simulink model "ame532Project1_Gimbal_Tracking_R2022aVersion_JeosUpdates"  (R2022a)
settings: Solver=ode4  StartTime=0.0  StopTime=35  FixedStep=0.1  RelTol=1e-3
model workspace (MAT data in the model file):
  theta : Simulink.Parameter (value not decoded)
values from neighbouring files (symbols this model uses):
  a0_s2 = 0    [AeroData.m]
  a0_s3 = 0    [AeroData.m]
  a0_s4 = 0.05    [AeroData.m]
  a0_s5 = 0.05    [AeroData.m]
  CD0_s2 = 0.01    [AeroData.m]
  CD0_s3 = 0.01    [AeroData.m]
  CD0_s4 = 0.01    [AeroData.m]
  CD0_s5 = 0.01    [AeroData.m]
  CDa_s2 = 1    [AeroData.m]
  CDa_s3 = 1    [AeroData.m]
  CDa_s4 = 1    [AeroData.m]
  CDa_s5 = 1    [AeroData.m]
  CL0_s2 = 0    [AeroData.m]
  CL0_s3 = 0    [AeroData.m]
  CL0_s4 = 0.05    [AeroData.m]
  CL0_s5 = 0.05    [AeroData.m]
  CM0_s2 = 0    [AeroData.m]
  CM0_s3 = 0    [AeroData.m]
  CM0_s4 = -0.05    [AeroData.m]
  CM0_s5 = -0.05    [AeroData.m]
  CMa_s2 = 0    [AeroData.m]
  CMa_s3 = 0    [AeroData.m]
  CMa_s4 = 0    [AeroData.m]
  CMa_s5 = 0    [AeroData.m]
  e_s2 = 0.8    [AeroData.m]
  e_s3 = 0.8    [AeroData.m]
  e_s4 = 0.9    [AeroData.m]
  e_s5 = 0.9    [AeroData.m]
  i_s2 = 0    [AeroData.m]
  i_s3 = 0    [AeroData.m]
  i_s4 = 0.05    [AeroData.m]
  i_s5 = 0.05    [AeroData.m]
  Jxx = 1    [Sim_sixDOFdriverScript.m]
  Jxy = 0.    (= 0)    [Sim_sixDOFdriverScript.m]
  Jxz = 3    [Sim_sixDOFdriverScript.m]
  Jyx = 2    [Sim_sixDOFdriverScript.m]
  Jyy = 2    [Sim_sixDOFdriverScript.m]
  Jyz = 0    [Sim_sixDOFdriverScript.m]
  Jzx = Jxz    (= 3)    [Sim_sixDOFdriverScript.m]
  Jzy = Jyz    (= 0)    [Sim_sixDOFdriverScript.m]
  Jzz = 2    [Sim_sixDOFdriverScript.m]
  LL = 0.8    [Sim_sixDOFdriverScript.m]
  MM = 0.8    [Sim_sixDOFdriverScript.m]
  n_s2 = [0; 0; -1]    [AeroData.m]
  n_s3 = [0; 1; 0]    [AeroData.m]
  n_s4 = [0; 0; -1]    [AeroData.m]
  n_s5 = [0; 0; -1]    [AeroData.m]
  NN = 0.8    [Sim_sixDOFdriverScript.m]
  rEarth = 6378100    [Sim_sixDOFdriverScript.m]
  ro = 1.225    [AeroData.m]
undefined symbols (not defined in the file or in its folder): AR_s2, AR_s3, AR_s4, AR_s5, area_s2, area_s3, area_s4, area_s5, c_s2, c_s3, c_s4, c_s5, earthRadius, x_S2_B_B, x_S3_B_B, x_S4_B_B, x_S5_B_B
libraries: simulink_extras x37, matrix_library x21, aerolibutil x6, aerolibfltsims x4, simulink x3, vrlib x2, aerolibtransform2 x2, sharedutil x2
(part 2 of 5)

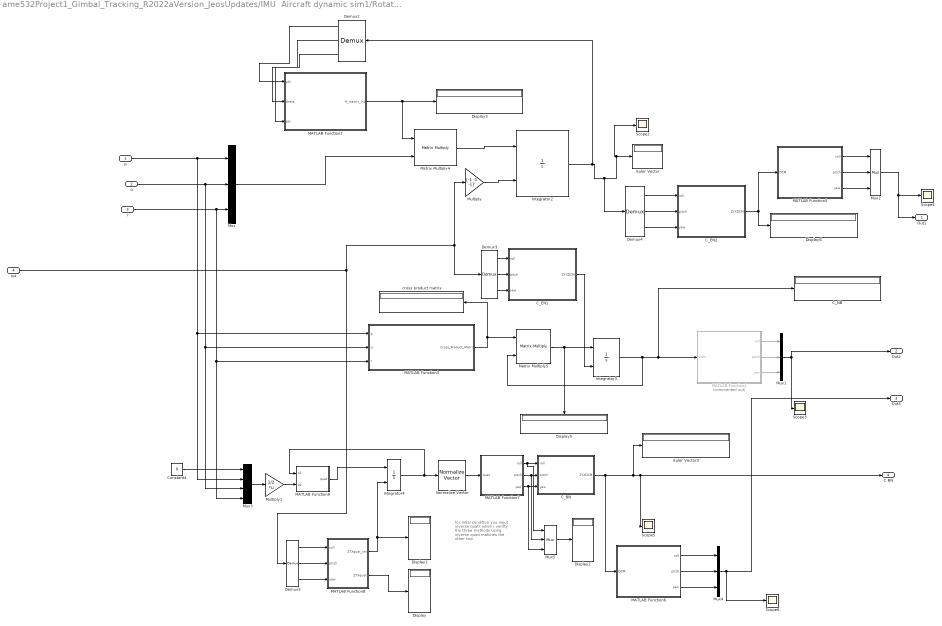
== system ame532Project1_Gimbal_Tracking_R2022aVersion_JeosUpdates/IMU  Aircraft dynamic sim1/Rotational Kinematics ==
  note: for intial condition you input inverse quat?
      | when I verifty the three methods using inverse quad matches the other two
  p : Inport
  q : Inport  Port=2
  r : Inport  Port=3
  In4 : Inport  Port=4
  C_BN : MATLAB Function  TreatAsAtomicUnit=on
  C_EN1 : MATLAB Function  TreatAsAtomicUnit=on
  C_EN2 : MATLAB Function  TreatAsAtomicUnit=on
  C_NB : Display
  Constant4 : Constant  Value=0
  Demux{2..5} (4 alike) : Demux  Outputs=3
  Display{,1..3,5..6} (6 alike) : Display
  Euler Vector : Display
  Euler Vector3 : Display
  Integrator2 : Integrator  InitialConditionSource=external
  Integrator3 : Integrator  InitialConditionSource=external
  Integrator4 : Integrator  InitialConditionSource=external  InitialCondition=[1 0 0 0]'
  MATLAB Function2 : MATLAB Function  TreatAsAtomicUnit=on
  MATLAB Function3 : MATLAB Function  TreatAsAtomicUnit=on
  MATLAB Function4 : MATLAB Function  Commented=on  TreatAsAtomicUnit=on
  MATLAB Function5 : MATLAB Function  TreatAsAtomicUnit=on
  MATLAB Function6 : MATLAB Function  TreatAsAtomicUnit=on
  MATLAB Function7 : MATLAB Function  TreatAsAtomicUnit=on
  MATLAB Function8 : MATLAB Function  TreatAsAtomicUnit=on
  MATLAB Function9 : MATLAB Function  TreatAsAtomicUnit=on
  Matrix Multiply4 : Product  Multiplication=Matrix(*)
  Matrix Multiply5 : Product  Multiplication=Matrix(*)
  Multiply : Gain  Gain=[-1 -1 -1]'
  Multiply1 : Gain  Gain=1/2  Multiplication=Matrix(K*u)
  Mux{,1..2,4..5} (5 alike) : Mux  Inputs=3
  Mux3 : Mux
  Normalize Vector : vrlib/Utilities/Normalize Vector  maxzero=0
  Scope{2..6} (5 alike) : Scope
  cross product matrix : Display
  Out1 : Outport
  Out2 : Outport  Port=2
  Out3 : Outport  Port=3
  C BN : Outport  Port=4
  wires:
  Matrix Multiply4/1 -> Integrator2/1
  In4/1 -> Multiply/1, Demux3/1, Demux5/1
  MATLAB Function4/3(yaw) -> Mux1/3
  Integrator2/1 -> Scope2/1, Euler Vector/1, Demux4/1, Demux2/1
  MATLAB Function2/1(H_matrix_inv) -> Display3/1, Matrix Multiply4/1
  MATLAB Function6/2(pitch) -> Mux4/2
  r/1 -> Mux3/4, MATLAB Function3/3(r), Mux/3
  Matrix Multiply5/1 -> Display5/1, Integrator3/1
  Mux/1 -> Matrix Multiply4/2
  q/1 -> Mux3/3, MATLAB Function3/2(q), Mux/2
  C_BN/1(ZYXDCM) -> MATLAB Function6/1(DCM), C BN/1, Scope5/1, Euler Vector3/1
  C_EN1/1(ZYXDCM) -> Integrator3/2
  MATLAB Function5/2(pitch) -> Mux2/2
  Mux1/1 -> Out2/1, Scope3/1
  MATLAB Function4/1(roll) -> Mux1/1
  Demux2/2 -> MATLAB Function2/2(theta)
  Demux4/3 -> C_EN2/3(yaw)
  MATLAB Function4/2(pitch) -> Mux1/2
  Demux2/3 -> MATLAB Function2/3(psi)
  Demux2/1 -> MATLAB Function2/1(phi)
  Demux5/1 -> MATLAB Function8/1(roll)
  Demux3/1 -> C_EN1/1(roll)
  Demux5/2 -> MATLAB Function8/2(pitch)
  Demux4/1 -> C_EN2/1(roll)
  Demux3/3 -> C_EN1/3(yaw)
  Multiply/1 -> Integrator2/2
  C_EN2/1(ZYXDCM) -> Display6/1, MATLAB Function5/1(DCM)
  Normalize Vector/1 -> MATLAB Function7/1(quat)
  MATLAB Function9/1(quat) -> Integrator4/1
  Integrator3/1 -> Matrix Multiply5/2, MATLAB Function4/1(DCM), C_NB/1
  p/1 -> Mux3/2, MATLAB Function3/1(p), Mux/1
  Integrator4/1 -> Normalize Vector/1, MATLAB Function9/1(q1)
  MATLAB Function7/3(yaw) -> Mux5/3, C_BN/3(yaw)
  Mux2/1 -> Out1/1, Scope4/1
  MATLAB Function5/3(yaw) -> Mux2/3
  Constant4/1 -> Mux3/1
  Mux3/1 -> Multiply1/1
  Mux4/1 -> Out3/1, Scope6/1
  MATLAB Function7/1(roll) -> Mux5/1, C_BN/1(roll)
  MATLAB Function5/1(roll) -> Mux2/1
  Demux5/3 -> MATLAB Function8/3(yaw)
  MATLAB Function6/1(roll) -> Mux4/1
  MATLAB Function6/3(yaw) -> Mux4/3
  Multiply1/1 -> MATLAB Function9/2(q2)
  MATLAB Function3/1(Cross_Product_Matrix) -> Matrix Multiply5/1, cross product matrix/1
  Demux4/2 -> C_EN2/2(pitch)
  Demux3/2 -> C_EN1/2(pitch)
  MATLAB Function7/2(pitch) -> Mux5/2, C_BN/2(pitch)
  MATLAB Function8/1(ZYXquat_inv) -> Integrator4/2, Display1/1
  MATLAB Function8/2(ZYXquat) -> Display/1
  Mux5/1 -> Display2/1

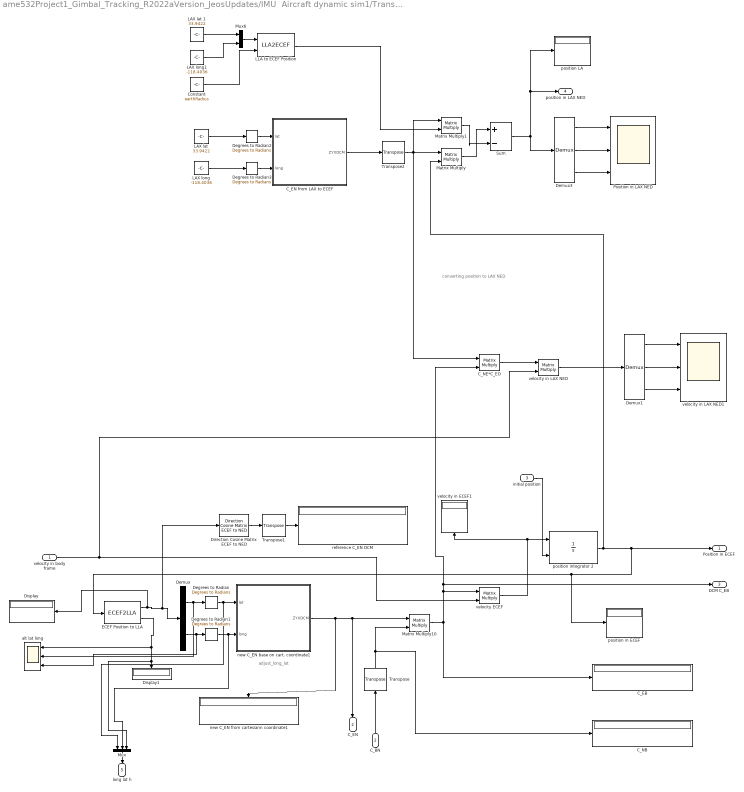
== system ame532Project1_Gimbal_Tracking_R2022aVersion_JeosUpdates/IMU  Aircraft dynamic sim1/Translational Kinematics ==
  note: converting position to LAX NED
  note: adjust_long_lat
  velocity in body frame : Inport
  C_BN : Inport  Port=2
  initial position : Inport  Port=3
  C_EB : Display
  C_EN from LAX to ECEF : MATLAB Function  TreatAsAtomicUnit=on
  C_NB : Display
  C_NE*C_EO : Product  Multiplication=Matrix(*)
  Constant : Constant  Value=earthRadius
  Degrees to Radian{,1..3} (4 alike) : simulink_extras/Transformations/Degrees to Radians
  Demux : Demux  Outputs=2
  Demux1 : Demux  Outputs=3
  Demux3 : Demux  Outputs=3
  Direction Cosine Matrix ECEF to NED : aerolibtransform2/Direction Cosine Matrix ECEF to NED
  Display : Display
  Display1 : Display
  ECEF Position to LLA : ECEF2LLA  ptype=Custom  R=earthRadius
  "LAX lat " : Constant  Value=33.9422
  LAX lat 1 : Constant  Value=33.9422
  LAX long : Constant  Value=-118.4036
  LAX long1 : Constant  Value=-118.4036
  LLA to ECEF Position : LLA2ECEF
  Matrix Multiply : Product  Multiplication=Matrix(*)
  Matrix Multiply1 : Product  Multiplication=Matrix(*)
  Matrix Multiply10 : Product  Multiplication=Matrix(*)
  Mux : Mux  Inputs=3
  Mux6 : Mux  Inputs=2
  Position in LAX NED : Scope  NumInputPorts=3
  Sum : Sum  Inputs=|+-
  Transpose : matrix_library/Transpose
  Transpose1 : matrix_library/Transpose
  Transpose2 : matrix_library/Transpose
  alt lat long : Scope  NumInputPorts=3
  new C_EN base on cart. coordinate1 : MATLAB Function  TreatAsAtomicUnit=on
  new C_EN from cartesiann coordinate1 : Display
  "position LA " : Display
  position in ECEF : Display
  position integrator 2 : Integrator  InitialConditionSource=external  InitialCondition=[6378100,0,0]'
  reference C_EN DCM : Display
  velocity ECEF : Product  Multiplication=Matrix(*)
  velocity in ECEF1 : Display
  velocity in LAX NED : Product  Multiplication=Matrix(*)
  velocity in LAX NED1 : Scope  NumInputPorts=3
  Position in ECEF : Outport
  C_EN : Outport  Port=2
  DCM C_EB : Outport  Port=3
  position in LAX NED : Outport  Port=4
  long lat h : Outport  Port=5
  wires:
  initial position/1 -> position integrator 2/2
  new C_EN base on cart. coordinate1/1(ZYXDCM) -> new C_EN from cartesiann coordinate1/1, C_EN/1, Matrix Multiply10/1
  Matrix Multiply10/1 -> C_EB/1, DCM C_EB/1, C_NE*C_EO/2, velocity ECEF/1
  velocity ECEF/1 -> position integrator 2/1, velocity in ECEF1/1
  velocity in body frame/1 -> velocity in LAX NED/2, velocity ECEF/2
  C_BN/1 -> Transpose/1
  ECEF Position to LLA/1 -> Direction Cosine Matrix ECEF to NED/1, Demux/1, Display/1
  ECEF Position to LLA/2 -> alt lat long/1, Mux/3, Display1/1
  Demux/1 -> Degrees to Radian/1, alt lat long/2
  Demux/2 -> alt lat long/3, Degrees to Radian1/1
  Degrees to Radian/1 -> Mux/1, new C_EN base on cart. coordinate1/1(lat)
  Degrees to Radian1/1 -> Mux/2, new C_EN base on cart. coordinate1/2(long)
  Transpose/1 -> C_NB/1, Matrix Multiply10/2
  Direction Cosine Matrix ECEF to NED/1 -> Transpose1/1
  Transpose1/1 -> reference C_EN DCM/1
  Mux/1 -> long lat h/1
  "LAX lat "/1 -> Degrees to Radian2/1
  LAX long/1 -> Degrees to Radian3/1
  Degrees to Radian2/1 -> C_EN from LAX to ECEF/1(lat)
  Degrees to Radian3/1 -> C_EN from LAX to ECEF/2(long)
  C_EN from LAX to ECEF/1(ZYXDCM) -> Transpose2/1
  Demux3/2 -> Position in LAX NED/2
  Demux3/3 -> Position in LAX NED/3
  Demux3/1 -> Position in LAX NED/1
  Transpose2/1 -> C_NE*C_EO/1, Matrix Multiply1/1, Matrix Multiply/1
  LAX long1/1 -> Mux6/2
  LAX lat 1/1 -> Mux6/1
  Constant/1 -> LLA to ECEF Position/2
  Mux6/1 -> LLA to ECEF Position/1
  LLA to ECEF Position/1 -> Matrix Multiply1/2
  Matrix Multiply/1 -> Sum/1
  Matrix Multiply1/1 -> Sum/2
  Sum/1 -> "position LA "/1, position in LAX NED/1, Demux3/1
  position integrator 2/1 -> Position in ECEF/1, ECEF Position to LLA/1, position in ECEF/1, Matrix Multiply/2
  C_NE*C_EO/1 -> velocity in LAX NED/1
  Demux1/2 -> velocity in LAX NED1/2
  velocity in LAX NED/1 -> Demux1/1
  Demux1/3 -> velocity in LAX NED1/3
  Demux1/1 -> velocity in LAX NED1/1

== system ame532Project1_Gimbal_Tracking_R2022aVersion_JeosUpdates/IMU  Aircraft dynamic sim1/Unused tranlational kinmatics ==
  In1 : Inport
  In2 : Inport  Port=2
  In3 : Inport  Port=3
  C_EN4 : MATLAB Function  TreatAsAtomicUnit=on
  DCM4 : Display
  Matrix Multiply8 : Product  Multiplication=Matrix(*)
  Matrix Multiply9 : Product  Multiplication=Matrix(*)
  Scope7 : Scope
  Transpose : matrix_library/Transpose
  pitch4 : Constant  Value=pi/2
  position integrator 1 : Integrator  InitialConditionSource=external  InitialCondition=[6378100,0,0]'
  position vector2 : Display
  roll4 : Constant  Value=0
  velocity in earth frame : Display
  yaw4 : Constant  Value=0
  wires:
  Matrix Multiply9/1 -> DCM4/1, Matrix Multiply8/1
  position integrator 1/1 -> Scope7/1, position vector2/1
  C_EN4/1(ZYXDCM) -> Matrix Multiply9/1
  Matrix Multiply8/1 -> velocity in earth frame/1, position integrator 1/1
  yaw4/1 -> C_EN4/3(yaw)
  pitch4/1 -> C_EN4/2(pitch)
  Transpose/1 -> Matrix Multiply9/2
  roll4/1 -> C_EN4/1(roll)
  In2/1 -> Matrix Multiply8/2
  In1/1 -> position integrator 1/2
  In3/1 -> Transpose/1

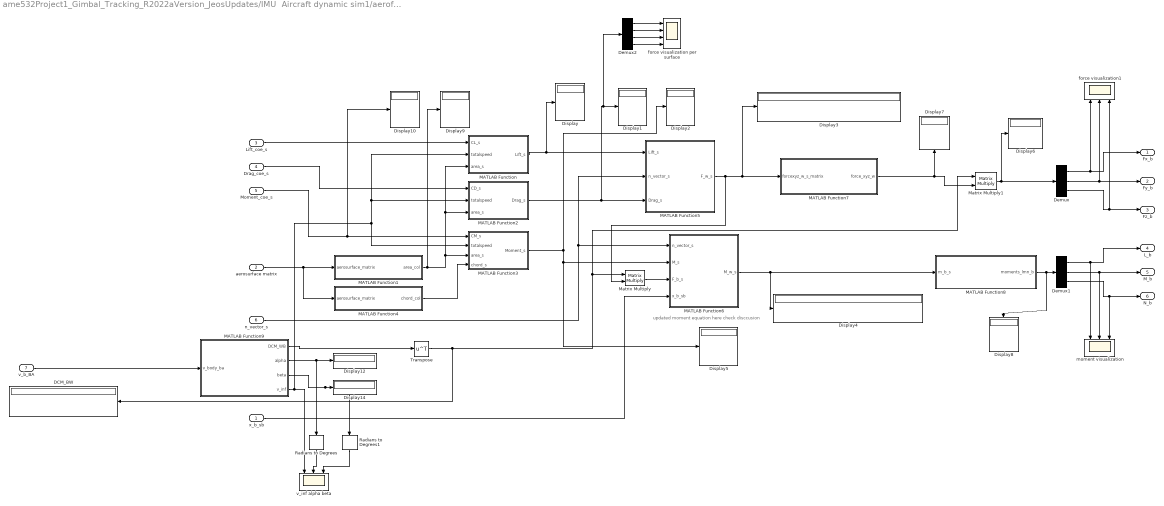
== system ame532Project1_Gimbal_Tracking_R2022aVersion_JeosUpdates/IMU  Aircraft dynamic sim1/aeroforce & moment block ==
  note: updated moment equation here check disccusion
  x_b_sb : Inport
  aerosurface matrix : Inport  Port=2
  Lift_coe_s : Inport  Port=3
  Drag_coe_s : Inport  Port=4
  Moment_coe_s : Inport  Port=5
  n_vector_s : Inport  Port=6
  v_b_BA : Inport  Port=7
  DCM_BW : Display
  Demux : Demux  Outputs=3
  Demux1 : Demux  Outputs=3
  Demux2 : Demux
  Display{,1..10,12,14} (13 alike) : Display
  MATLAB Function : MATLAB Function  TreatAsAtomicUnit=on
  MATLAB Function1 : MATLAB Function  TreatAsAtomicUnit=on
  MATLAB Function2 : MATLAB Function  TreatAsAtomicUnit=on
  MATLAB Function3 : MATLAB Function  TreatAsAtomicUnit=on
  MATLAB Function4 : MATLAB Function  TreatAsAtomicUnit=on
  MATLAB Function5 : MATLAB Function  TreatAsAtomicUnit=on
  MATLAB Function6 : MATLAB Function  TreatAsAtomicUnit=on
  MATLAB Function7 : MATLAB Function  TreatAsAtomicUnit=on
  MATLAB Function8 : MATLAB Function  TreatAsAtomicUnit=on
  MATLAB Function9 : MATLAB Function  TreatAsAtomicUnit=on
  Matrix Multiply : Product  Multiplication=Matrix(*)
  Matrix Multiply1 : Product  Multiplication=Matrix(*)
  Radians to Degrees : simulink_extras/Transformations/Radians to Degrees
  Radians to Degrees1 : simulink_extras/Transformations/Radians to Degrees
  Transpose : Math  Operator=transpose
  force visualization per surface : Scope  NumInputPorts=4
  force visualization1 : Scope  NumInputPorts=3
  moment visualization : Scope  NumInputPorts=3
  v_inf alpha beta : Scope  NumInputPorts=3
  Fx_b : Outport
  Fy_b : Outport  Port=2
  Fz_b : Outport  Port=3
  L_b : Outport  Port=4
  M_b : Outport  Port=5
  N_b : Outport  Port=6
  wires:
  Lift_coe_s/1 -> MATLAB Function/1(CL_s)
  MATLAB Function9/4(v_inf) -> v_inf alpha beta/1, MATLAB Function2/2(totalspeed), MATLAB Function/2(totalspeed), MATLAB Function3/2(totalspeed)
  aerosurface matrix/1 -> MATLAB Function4/1(aerosurface_matrix), MATLAB Function1/1(aerosurface_matrix)
  MATLAB Function1/1(area_col) -> Display9/1, MATLAB Function2/3(area_s), MATLAB Function/3(area_s), MATLAB Function3/3(area_s)
  Drag_coe_s/1 -> MATLAB Function2/1(CD_s)
  Moment_coe_s/1 -> Display10/1, MATLAB Function3/1(CM_s)
  MATLAB Function4/1(chord_col) -> MATLAB Function3/4(chord_s)
  n_vector_s/1 -> MATLAB Function5/2(n_vector_s), MATLAB Function6/1(n_vector_s)
  MATLAB Function/1(Lift_s) -> Display/1, MATLAB Function5/1(Lift_s)
  MATLAB Function2/1(Drag_s) -> MATLAB Function5/3(Drag_s), Demux2/1, Display1/1
  MATLAB Function3/1(Moment_s) -> Display5/1, MATLAB Function6/2(M_s), Display2/1
  MATLAB Function6/1(M_w_s) -> Display4/1, MATLAB Function8/1(m_b_s)
  Matrix Multiply/1 -> MATLAB Function6/3(F_b_s)
  x_b_sb/1 -> MATLAB Function6/4(x_b_sb)
  MATLAB Function5/1(F_w_s) -> Matrix Multiply/2, Display3/1, MATLAB Function7/1(forcexyz_w_s_matrix)
  MATLAB Function7/1(force_xyz_w) -> Matrix Multiply1/2, Display7/1
  MATLAB Function8/1(moments_lmn_b) -> Demux1/1, Display8/1
  Matrix Multiply1/1 -> Demux/1, Display6/1
  MATLAB Function9/1(DCM_WB) -> Transpose/1
  v_b_BA/1 -> MATLAB Function9/1(v_body_ba)
  MATLAB Function9/2(alpha) -> Radians to Degrees/1, Display12/1
  MATLAB Function9/3(beta) -> Display14/1, Radians to Degrees1/1
  Demux1/1 -> L_b/1, moment visualization/1
  Demux1/2 -> M_b/1, moment visualization/2
  Demux1/3 -> moment visualization/3, N_b/1
  Demux/1 -> Fx_b/1, force visualization1/1
  Demux/2 -> Fy_b/1, force visualization1/2
  Demux/3 -> Fz_b/1, force visualization1/3
  Transpose/1 -> Matrix Multiply1/1, Matrix Multiply/1, DCM_BW/1
  Radians to Degrees/1 -> v_inf alpha beta/2
  Radians to Degrees1/1 -> v_inf alpha beta/3
  Demux2/4 -> force visualization per surface/4
  Demux2/3 -> force visualization per surface/3
  Demux2/2 -> force visualization per surface/2
  Demux2/1 -> force visualization per surface/1

== system ame532Project1_Gimbal_Tracking_R2022aVersion_JeosUpdates/IMU  Aircraft dynamic sim1/aeroforce coefficient block ==
  note: next step is to create lift force, CD, CM
  aero surface property matrix : Inport
  real wind in N axes : Inport  Port=2
  velocity in bodyframe : Inport  Port=3
  C_BN : Inport  Port=4
  CD0 : Constant  Value=[0.01 0.01 0.01 0.01]'
  CD1 : Constant  Value=[0.9 0.9 0.8 0.8]'
  CD_a : Constant  Value=[1 1 1 1]'
  CL over time : Scope  NumInputPorts=4
  CL0 : Constant  Value=[0.05 0.05 0 0]'
  CM_0 : Constant  Value=[-0.05 -0.05 0 0]'
  CM_a : Constant  Value=[0 0 0 0]'
  Demux1 : Demux
  Demux5 : Demux
  Demux6 : Demux  Outputs=3
  Display{,1..3,5..7} (7 alike) : Display
  MATLAB Function : MATLAB Function  TreatAsAtomicUnit=on
  MATLAB Function1 : MATLAB Function  TreatAsAtomicUnit=on
  MATLAB Function2 : MATLAB Function  TreatAsAtomicUnit=on
  MATLAB Function3 : MATLAB Function  TreatAsAtomicUnit=on
  alpha : Scope  NumInputPorts=4
  alpha_0 : Constant  Value=[0.05 0.05 0 0]'
  calculatie alpha : MATLAB Function  TreatAsAtomicUnit=on
  extract matrix function : MATLAB Function  TreatAsAtomicUnit=on
  extract matrix function1 : MATLAB Function  TreatAsAtomicUnit=on
  i0 : Constant  Value=[0.05 0.05 0 0]'
  n vector(4 5 2 3 from left to right) : Constant  Value=[0 0 0 0;0 0 0 1;-1 -1 -1 0]
  velocity in body wrt air : Scope  NumInputPorts=3
  Lift coefficient_s : Outport
  Drag coefficient_s : Outport  Port=2
  Moment coefficient_s : Outport  Port=3
  n_vector_s : Outport  Port=4
  v_B_BA : Outport  Port=5
  wires:
  aero surface property matrix/1 -> extract matrix function1/1(aero_surface_matrix), extract matrix function/1(aero_surface_matrix)
  extract matrix function/1(AR_matrix) -> Display/1, MATLAB Function/1(AR_matrix)
  MATLAB Function/1(CL_a) -> MATLAB Function1/2(CL_a), Display1/1
  n vector(4 5 2 3 from left to right)/1 -> n_vector_s/1, calculatie alpha/3(n_vector)
  velocity in bodyframe/1 -> calculatie alpha/2(v_B)
  i0/1 -> calculatie alpha/1(i0)
  CL0/1 -> MATLAB Function1/1(CL0)
  Demux5/2 -> CL over time/2
  Demux5/1 -> CL over time/1
  Demux5/3 -> CL over time/3
  MATLAB Function1/1(CL_s) -> Demux5/1, Display3/1, Lift coefficient_s/1, MATLAB Function2/5(CL_s)
  Demux5/4 -> CL over time/4
  real wind in N axes/1 -> calculatie alpha/4(wind_w)
  extract matrix function1/1(AR_matrix) -> MATLAB Function2/7(AR)
  CD1/1 -> MATLAB Function2/6(e)
  alpha_0/1 -> MATLAB Function2/3(alpha_0)
  CD0/1 -> MATLAB Function2/1(CD_0)
  CD_a/1 -> MATLAB Function2/2(CD_a)
  MATLAB Function2/1(CD_s) -> Drag coefficient_s/1, Display6/1
  CM_0/1 -> MATLAB Function3/2(CM_0)
  CM_a/1 -> MATLAB Function3/3(CM_a)
  MATLAB Function3/1(CM_s) -> Moment coefficient_s/1, Display7/1
  C_BN/1 -> calculatie alpha/5(C_BN)
  calculatie alpha/2(v_B_BA) -> Demux6/1, Display5/1, v_B_BA/1
  Demux6/3 -> velocity in body wrt air/3
  Demux6/2 -> velocity in body wrt air/2
  Demux6/1 -> velocity in body wrt air/1
  Demux1/1 -> alpha/1
  Demux1/2 -> alpha/2
  Demux1/3 -> alpha/3
  Demux1/4 -> alpha/4
  calculatie alpha/1(alpha) -> MATLAB Function3/1(alpha), MATLAB Function2/4(alpha), MATLAB Function1/3(alpha), Display2/1, Demux1/1

== system ame532Project1_Gimbal_Tracking_R2022aVersion_JeosUpdates/IMU  Aircraft dynamic sim1/mass & aero property calculation ==
  u : Inport
  CG calculation : MATLAB Function  TreatAsAtomicUnit=on
  Display : Display
  Display1 : Display
  J matrix : Display
  MATLAB Function : MATLAB Function  TreatAsAtomicUnit=on
  MATLAB Function1 : MATLAB Function  TreatAsAtomicUnit=on
  MATLAB Function2 : MATLAB Function  TreatAsAtomicUnit=on
  Mux : Mux  Inputs=3
  Submatrix : matrix_library/Submatrix  RowSpan=All rows  RowStartMode=First  RowStartIndex=1  RowEndMode=Last  RowEndIndex=1  ColSpan=One column  ColStartMode=First  ColStartIndex=1  ColEndMode=Last  ColEndIndex=1
  Sum of Elements : Sum  Inputs=+
  aero prop matrix x y z c b A AR : Display
  m matrix : Display
  x_b_sb : Display
  total mass : Outport
  cg coordinate : Outport  Port=2
  J_matrix : Outport  Port=3
  aero surface property matrix : Outport  Port=4
  x b sb : Outport  Port=5
  wires:
  CG calculation/1(cg_x) -> Mux/1
  u/1 -> MATLAB Function1/2(m_matrix), MATLAB Function2/1(M_matrix), m matrix/1, Submatrix/1, MATLAB Function/2(M_matrix), CG calculation/1(M_matrix)
  CG calculation/2(cg_y) -> Mux/2
  CG calculation/3(cg_z) -> Mux/3
  Mux/1 -> MATLAB Function1/3(cg_location), MATLAB Function/1(cg_location), cg coordinate/1, Display/1
  Submatrix/1 -> Sum of Elements/1
  Sum of Elements/1 -> total mass/1, Display1/1
  MATLAB Function/1(J_matrix) -> J_matrix/1, J matrix/1
  MATLAB Function2/1(aero_prop) -> MATLAB Function1/1(aero_prop_matrix), aero prop matrix x y z c b A AR/1, aero surface property matrix/1
  MATLAB Function1/1(x_b_s_ac) -> x b sb/1, x_b_sb/1

== system ame532Project1_Gimbal_Tracking_R2022aVersion_JeosUpdates/IMU  Aircraft dynamic sim1/measurement subsystem ==
  velocity in body frame : Inport
  Asin : Trigonometry  Operator=asin
  Atan2 : Trigonometry  Operator=atan2
  Demux : Demux  Outputs=3
  Demux1 : Demux  Outputs=3
  Display : Display
  Divide : Product  Inputs=*/  RndMeth=Zero  SaturateOnIntegerOverflow=on
  MATLAB Function : MATLAB Function  TreatAsAtomicUnit=on
  Mux : Mux  Inputs=3
  Radians to Degrees{,1..3} (4 alike) : simulink_extras/Transformations/Radians to Degrees
  v_inf alpha beta : Scope  NumInputPorts=3
  total speed : Outport
  alpha (AoA) : Outport  Port=2
  beta (side slip) : Outport  Port=3
  wires:
  MATLAB Function/1(magnitude) -> Divide/2, Mux/1, total speed/1, v_inf alpha beta/1
  velocity in body frame/1 -> MATLAB Function/1(velocity), Demux1/1, Demux/1
  Demux/3 -> Atan2/1
  Demux/1 -> Atan2/2
  Atan2/1 -> alpha (AoA)/1, Radians to Degrees2/1, Radians to Degrees/1
  Demux1/2 -> Divide/1
  Divide/1 -> Asin/1
  Asin/1 -> beta (side slip)/1, Radians to Degrees3/1, Radians to Degrees1/1
  Mux/1 -> Display/1
  Radians to Degrees/1 -> Mux/2
  Radians to Degrees1/1 -> Mux/3
  Radians to Degrees2/1 -> v_inf alpha beta/2
  Radians to Degrees3/1 -> v_inf alpha beta/3

== system ame532Project1_Gimbal_Tracking_R2022aVersion_JeosUpdates/IMU  Aircraft dynamic sim1/rotational dynamics ==
  note: body rate acceleration
  J_matrix : Inport
  Initial w : Inport  Port=2
  moment in body : Inport  Port=3
  Cross Product : matrix_library/Cross Product
  Display4 : Display
  Display5 : Display
  Display6 : Display
  Invert 3x3 Matrix : aerolibutil/Invert  3x3 Matrix
  Matrix Multiply4 : Product  Multiplication=Matrix(*)
  Matrix Multiply5 : Product  Multiplication=Matrix(*)
  Sum : Sum  Inputs=|+-
  body rate : Integrator  InitialConditionSource=external  InitialCondition=[0 0 0]'
  omega_b : Outport
  wires:
  Cross Product/1 -> Sum/2, Display6/1
  Sum/1 -> Matrix Multiply4/2
  J_matrix/1 -> Matrix Multiply5/1, Invert 3x3 Matrix/1
  body rate/1 -> omega_b/1, Matrix Multiply5/2, Cross Product/1
  Matrix Multiply4/1 -> Display5/1, body rate/1
  Invert 3x3 Matrix/1 -> Matrix Multiply4/1, Display4/1
  Matrix Multiply5/1 -> Cross Product/2
  Initial w/1 -> body rate/2
  moment in body/1 -> Sum/1

== system ame532Project1_Gimbal_Tracking_R2022aVersion_JeosUpdates/IMU  Aircraft dynamic sim1/translational dynamics ==
  note: counter gravity before needs to be accounted by a DCM
  note: velocity in body frame
  note: acceleration in body frame
  p : Inport
  q : Inport  Port=2
  r : Inport  Port=3
  ZYXDCM : Inport  Port=4
  external forces : Inport  Port=5
  intial velocity : Inport  Port=6
  Display{,1..4,8..9} (7 alike) : Display
  Integrator5 : Integrator  InitialConditionSource=external
  MATLAB Function10 : MATLAB Function  TreatAsAtomicUnit=on
  Matrix Multiply6 : Product  Multiplication=Matrix(*)
  Matrix Multiply7 : Product  Multiplication=Matrix(*)
  Scope : Scope
  Sum : Sum  Inputs=|++-
  gravity in N_frame : Constant  Value=[0 0 9.81]'
  weight : Gain  Gain=1/0.48
  velocity in body frame : Outport
  wires:
  MATLAB Function10/1(Cross_Product_Matrix) -> Matrix Multiply7/1, Display8/1
  Integrator5/1 -> velocity in body frame/1, Display1/1, Matrix Multiply7/2
  Sum/1 -> Display3/1, Scope/1, Integrator5/1
  Matrix Multiply6/1 -> Sum/2, Display2/1
  Matrix Multiply7/1 -> Sum/3, Display9/1
  ZYXDCM/1 -> Display/1, Matrix Multiply6/1
  q/1 -> MATLAB Function10/2(q)
  p/1 -> MATLAB Function10/1(p)
  r/1 -> MATLAB Function10/3(r)
  intial velocity/1 -> Integrator5/2
  gravity in N_frame/1 -> Matrix Multiply6/2
  external forces/1 -> weight/1
  weight/1 -> Sum/1, Display4/1

== system ame532Project1_Gimbal_Tracking_R2022aVersion_JeosUpdates/JeoIMUmodel/New Version ==
  LAX Initial Position : Inport
  Aero Forces and Moments : Subsystem
  Gyroscope : Subsystem
  Initial Body Rates PQR : Constant  Value=[0 0 0]'
  Integrator : Integrator  InitialConditionSource=external
  Manual Switch1 : ManualSwitch  CurrentSetting=0
  Rotational Dynamics : Subsystem
  Rotational Kinematics_Quaternions : Subsystem  Commented=on
  Rotational Kinematics_Strapdown : Subsystem  Commented=on
  Terminator : Terminator
  Terminator1 : Terminator
  TransKin_RotKin_TansDynam : Subsystem
  Position in LAX NED : Outport
  ECEF Position : Outport  Port=2
  DCM C_EB : Outport  Port=3
  wires:
  Aero Forces and Moments/2(Fext_B) -> TransKin_RotKin_TansDynam/2(Aero Forces)
  Initial Body Rates PQR/1 -> Integrator/2
  Aero Forces and Moments/1(Mext_B) -> Rotational Dynamics/2(Aero Moment)
  Gyroscope/1(Measured Body Rates) -> Manual Switch1/1  "Measured Body Rates"
  TransKin_RotKin_TansDynam/2(E_x_B_E_E) -> ECEF Position/1, Terminator1/1  "Position of Body from ECEF w.r.t ECEF attached to ECEF"
  Manual Switch1/1 -> TransKin_RotKin_TansDynam/1(wBodyRates_PQR)
  Rotational Dynamics/1(wdotVector Body Rates_PQR) -> Integrator/1  "wdotVector Body Rates_PQR"
  Integrator/1 -> Gyroscope/1(True Body Rates), Manual Switch1/2, Rotational Dynamics/1(wVector Body Rates_PQR)  "wVector Body Rates_PQR"
  TransKin_RotKin_TansDynam/3(V_B_E_B) -> Aero Forces and Moments/1(V_B_E_B)
  TransKin_RotKin_TansDynam/4(C_B_N) -> Aero Forces and Moments/2(C_B_N)
  TransKin_RotKin_TansDynam/1(Altitude_m) -> Terminator/1  "Distance of body from Earth Center (m)"
  LAX Initial Position/1 -> TransKin_RotKin_TansDynam/3(LAX Initial Pos)
  TransKin_RotKin_TansDynam/5(c_EB) -> DCM C_EB/1
  TransKin_RotKin_TansDynam/6(Position in LAX NED) -> Position in LAX NED/1

== system ame532Project1_Gimbal_Tracking_R2022aVersion_JeosUpdates/JeoIMUmodel/Old Version ==
  LAx Inital Pos : Inport
  Aero Forces and Moments : Subsystem
  Initial Body w Rates : Concatenate  NumInputs=3
  Integrator : Integrator  InitialConditionSource=external
  Manual Switch : ManualSwitch  CurrentSetting=0
  Pitch_rad/s : Constant  Value=0
  Roll_rad/s : Constant  Value=0
  Rotational Dynamics : Subsystem
  Rotational Kinematics_Quaternions : Subsystem  Commented=on
  Rotational Kinematics_Strapdown : Subsystem  Commented=on
  Terminator : Terminator
  Terminator1 : Terminator
  To Workspace : ToWorkspace  VariableName=yout  SaveFormat=Timeseries  SampleTime=-1
  TransKin_RotKin_TansDynam : Subsystem
  Vector Concatenate : Concatenate  NumInputs=3  Mode=Multidimensional array
  Yaw_rad/s : Constant  Value=0
  pitchRate_degPs : Constant  Value=0
  rollRate_degPs : Constant  Value=0
  yawRate_degPs : Constant
  Position in LAX NED : Outport
  ECEF Position : Outport  Port=2
  DCM C_EB : Outport  Port=3
  wires:
  Roll_rad/s/1 -> Initial Body w Rates/1
  Aero Forces and Moments/1(Mext_B) -> Rotational Dynamics/2(Aero Moment)
  Integrator/1 -> Manual Switch/2, Rotational Dynamics/1(wVector Body Rates_PQR)  "wVector Body Rates_PQR"
  TransKin_RotKin_TansDynam/4(C_B_N) -> Aero Forces and Moments/2(C_B_N)
  TransKin_RotKin_TansDynam/2(E_x_B_E_E) -> ECEF Position/1, Terminator1/1, To Workspace/1  "Position of Body from ECEF w.r.t ECEF attached to ECEF"
  pitchRate_degPs/1 -> Vector Concatenate/2
  TransKin_RotKin_TansDynam/5(c_EB) -> DCM C_EB/1
  TransKin_RotKin_TansDynam/1(Altitude_m) -> Terminator/1  "Distance of body from Earth Center (m)"
  Vector Concatenate/1 -> Manual Switch/1  "wVector Body Rates_PQR"
  yawRate_degPs/1 -> Vector Concatenate/3
  Pitch_rad/s/1 -> Initial Body w Rates/2
  Yaw_rad/s/1 -> Initial Body w Rates/3
  Rotational Dynamics/1(wdotVector Body Rates_PQR) -> Integrator/1  "wdotVector Body Rates_PQR"
  Aero Forces and Moments/2(Fext_B) -> TransKin_RotKin_TansDynam/2(Aero Forces)
  Initial Body w Rates/1 -> Integrator/2
  rollRate_degPs/1 -> Vector Concatenate/1
  TransKin_RotKin_TansDynam/6(position in LAX NED) -> Position in LAX NED/1
  Manual Switch/1 -> TransKin_RotKin_TansDynam/1(wBodyRates_PQR)
  TransKin_RotKin_TansDynam/3(V_B_E_B) -> Aero Forces and Moments/1(V_B_E_B)
  LAx Inital Pos/1 -> TransKin_RotKin_TansDynam/3(LAx Inital Pos)

== system ame532Project1_Gimbal_Tracking_R2022aVersion_JeosUpdates/JeoIMUmodel/New Version/Aero Forces and Moments ==
  V_B_E_B : Inport
  C_B_N : Inport  Port=2
  F&M Horiz Stab Surface (S2) : Subsystem
  F&M Horiz Stab Surface (S3) : Subsystem
  F&M Right Wing and Servo Surface (S4) : Subsystem
  F&M Right Wing and Servo Surface (S5) : Subsystem
  Matrix Multiply : Product  Multiplication=Matrix(*)
  Sum : Sum  Inputs=|+-
  Sum1 : Sum  Inputs=|++++
  Sum2 : Sum  Inputs=|++++
  Velocity of Air Mass w.r.t. NED as measured in NED : Concatenate  NumInputs=3
  Wind in Down Direction : Constant  Value=0
  Wind in East Direction : Constant  Value=0
  Wind in North Direction : Constant  Value=0
  Mext_B : Outport
  Fext_B : Outport  Port=2
  wires:
  V_B_E_B/1 -> F&M Right Wing and Servo Surface (S5)/1(v_B_E_B), F&M Right Wing and Servo Surface (S4)/1(v_B_E_B), F&M Horiz Stab Surface (S2)/1(v_B_E_B), F&M Horiz Stab Surface (S3)/1(v_B_E_B), Sum/1
  Velocity of Air Mass w.r.t. NED as measured in NED/1 -> Matrix Multiply/2  "V_A_N_N"
  Wind in North Direction/1 -> Velocity of Air Mass w.r.t. NED as measured in NED/1
  Wind in East Direction/1 -> Velocity of Air Mass w.r.t. NED as measured in NED/2
  Wind in Down Direction/1 -> Velocity of Air Mass w.r.t. NED as measured in NED/3
  Sum/1 -> F&M Horiz Stab Surface (S2)/2(V_B_A_B (Relative AIr Speed)), F&M Horiz Stab Surface (S3)/2(V_B_A_B (Relative AIr Speed)), F&M Right Wing and Servo Surface (S5)/2(V_B_A_B (Relative AIr Speed)), F&M Right Wing and Servo Surface (S4)/2(V_B_A_B (Relative AIr Speed))  "V_B_A_B (Relative AIr Speed)"
  F&M Horiz Stab Surface (S2)/2(LiftAndDragForceS2_B) -> Sum1/1
  F&M Horiz Stab Surface (S3)/2(LiftAndDragForceS3_B) -> Sum1/2
  F&M Right Wing and Servo Surface (S4)/2(LiftAndDragForceS4_B) -> Sum1/3
  F&M Right Wing and Servo Surface (S5)/2(LiftAndDragForceS5_B) -> Sum1/4
  Sum1/1 -> Fext_B/1
  F&M Horiz Stab Surface (S2)/1(momS2_B) -> Sum2/1
  F&M Horiz Stab Surface (S3)/1(momS3_B) -> Sum2/2
  F&M Right Wing and Servo Surface (S4)/1(momS4_B) -> Sum2/3
  F&M Right Wing and Servo Surface (S5)/1(momS5_B) -> Sum2/4
  Sum2/1 -> Mext_B/1
  C_B_N/1 -> Matrix Multiply/1
  Matrix Multiply/1 -> Sum/2  "V_A_N_B"

== system ame532Project1_Gimbal_Tracking_R2022aVersion_JeosUpdates/JeoIMUmodel/New Version/Gyroscope ==
  True Body Rates : Inport
  Band-Limited White Noise : simulink/Sources/Band-Limited White Noise  Commented=on  Cov=[0.1]  Ts=0.1  seed=[23341]
  Gyro Constant Bias : Constant  Value=0
  Gyro Scale Factor : Gain
  Sum : Sum  Inputs=|++
  Sum1 : Sum  Inputs=|++
  Measured Body Rates : Outport
  wires:
  True Body Rates/1 -> Sum/1
  Gyro Constant Bias/1 -> Sum/2
  Sum/1 -> Gyro Scale Factor/1
  Gyro Scale Factor/1 -> Sum1/1
  Band-Limited White Noise/1 -> Sum1/2
  Sum1/1 -> Measured Body Rates/1

== system ame532Project1_Gimbal_Tracking_R2022aVersion_JeosUpdates/JeoIMUmodel/New Version/Rotational Dynamics ==
  wVector Body Rates_PQR : Inport
  Aero Moment : Inport  Port=2
  Invert 3x3 Matrix : aerolibutil/Invert  3x3 Matrix
  Jmat : sharedutil/Create 3x3 Matrix  aMode=aMode
  Jxx : Constant  Value=Jxx
  Jxy : Constant  Value=Jxy
  Jxz : Constant  Value=Jxz
  Jyx : Constant  Value=Jyx
  Jyy : Constant  Value=Jyy
  Jyz : Constant  Value=Jyz
  Jzx : Constant  Value=Jzx
  Jzy : Constant  Value=Jzy
  Jzz : Constant  Value=Jzz
  Manual Switch : ManualSwitch
  Manual Switch1 : ManualSwitch  CurrentSetting=0
  Matrix Multiply2 : Product  Multiplication=Matrix(*)
  Pitch Body Moment : Constant  Value=MM
  Roll Body Moment : Constant  Value=LL
  Sum : Sum  Inputs=|+-
  Using Cross Product Matrix : Subsystem
  Using Cross Product Operator Only : Subsystem
  Vector Concatenate : Concatenate  NumInputs=3
  Yaw Body Moment : Constant  Value=NN
  wdotVector Body Rates_PQR : Outport
  wires:
  wVector Body Rates_PQR/1 -> Using Cross Product Operator Only/1(wPQR), Using Cross Product Matrix/1(wPQR)
  Jmat/1 -> Using Cross Product Matrix/2(J Matrix), Using Cross Product Operator Only/2(J Matrix), Invert 3x3 Matrix/1
  Using Cross Product Matrix/1(OmegaJw) -> Manual Switch1/1  "OmegaJw [3x1]"
  Sum/1 -> Matrix Multiply2/2
  Matrix Multiply2/1 -> wdotVector Body Rates_PQR/1
  Jxx/1 -> Jmat/1
  Jxy/1 -> Jmat/2
  Jxz/1 -> Jmat/3
  Jyx/1 -> Jmat/4
  Jyy/1 -> Jmat/5
  Jyz/1 -> Jmat/6
  Jzx/1 -> Jmat/7
  Jzy/1 -> Jmat/8
  Jzz/1 -> Jmat/9
  Invert 3x3 Matrix/1 -> Matrix Multiply2/1  "Jinv"
  Roll Body Moment/1 -> Vector Concatenate/1
  Pitch Body Moment/1 -> Vector Concatenate/2
  Yaw Body Moment/1 -> Vector Concatenate/3
  Vector Concatenate/1 -> Manual Switch/2  "Mext_B"
  Aero Moment/1 -> Manual Switch/1
  Manual Switch/1 -> Sum/1
  Manual Switch1/1 -> Sum/2
  Using Cross Product Operator Only/1(OmegaJw) -> Manual Switch1/2

== system ame532Project1_Gimbal_Tracking_R2022aVersion_JeosUpdates/JeoIMUmodel/New Version/Rotational Kinematics_Quaternions ==
  wVectorBodyRates_PQR : Inport
  Constant : Constant  Value=0
  Gain : Gain  Gain=0.5
  Integrator : Integrator
  Mux : Mux  Inputs=3
  NormalizeQuaternion : MATLAB Function  TreatAsAtomicUnit=on
  Quaternion Multiplication : aerolibutil/Quaternion Multiplication
  Vector Concatenate : Concatenate
  quaternionMultiplication : MATLAB Function  Commented=on  TreatAsAtomicUnit=on
  quaternionToeuler : MATLAB Function  TreatAsAtomicUnit=on
  Theta Vector_deg : Outport
  wires:
  wVectorBodyRates_PQR/1 -> Gain/1
  Gain/1 -> Vector Concatenate/2
  Constant/1 -> Vector Concatenate/1
  Integrator/1 -> NormalizeQuaternion/1(qin), quaternionToeuler/1(qin)  "q_B_N"
  quaternionToeuler/3(roll_deg) -> Mux/1
  quaternionToeuler/2(pitch_deg) -> Mux/2
  quaternionToeuler/1(yaw_deg) -> Mux/3
  NormalizeQuaternion/1(qoutNorm) -> Quaternion Multiplication/1  "q_B_N"
  Mux/1 -> Theta Vector_deg/1
  Quaternion Multiplication/1 -> Integrator/1
  Vector Concatenate/1 -> Quaternion Multiplication/2

== system ame532Project1_Gimbal_Tracking_R2022aVersion_JeosUpdates/JeoIMUmodel/New Version/Rotational Kinematics_Strapdown ==
  wVectorBodyRates_PQR : Inport
  Demux : Demux  Outputs=3
  Integrator : Integrator
  MatrixMultiply : Product  Multiplication=Matrix(*)
  Mux : Mux  Inputs=3
  Omega_B_N : MATLAB Function  TreatAsAtomicUnit=on
  dcmTOeuler : MATLAB Function  TreatAsAtomicUnit=on
  Theta Vector_deg : Outport
  wires:
  wVectorBodyRates_PQR/1 -> Demux/1
  Demux/1 -> Omega_B_N/1(P_degPs)
  Demux/2 -> Omega_B_N/2(Q_degPs)
  Demux/3 -> Omega_B_N/3(R_degPs)
  Omega_B_N/1(y) -> MatrixMultiply/1  "omega_B_N"
  MatrixMultiply/1 -> Integrator/1  "cdot_N_B"
  Integrator/1 -> MatrixMultiply/2, dcmTOeuler/1(inputDCM)  "c_N_B"
  dcmTOeuler/3(roll_deg) -> Mux/1
  dcmTOeuler/2(pitch_deg) -> Mux/2
  dcmTOeuler/1(yaw_deg) -> Mux/3
  Mux/1 -> Theta Vector_deg/1  "Theta Vector_deg"

== system ame532Project1_Gimbal_Tracking_R2022aVersion_JeosUpdates/JeoIMUmodel/New Version/TransKin_RotKin_TansDynam ==
  wBodyRates_PQR : Inport
  Aero Forces : Inport  Port=2
  LAX Initial Pos : Inport  Port=3
  E_xdot_B_E_B_xComp : Constant  Value=150
  E_xdot_B_E_B_yComp : Constant  Value=0
  E_xdot_B_E_B_zComp : Constant  Value=0
  Matrix Multiply : Product  Multiplication=Matrix(*)
  Mux2 : Mux  Inputs=3
  Pitch2_rad : Constant  Value=0
  Roll2_rad : Constant  Value=0
  Rotational Kinematics_Euler : Subsystem
  Translational Dynamics : Subsystem
  Translational Kinematics : Subsystem
  Transpose : Math  Operator=transpose
  Vector Concatenate : Concatenate  NumInputs=3
  Yaw2_rad : Constant  Value=0
  Altitude_m : Outport
  E_x_B_E_E : Outport  Port=2
  V_B_E_B : Outport  Port=3
  C_B_N : Outport  Port=4
  c_EB : Outport  Port=5
  Position in LAX NED : Outport  Port=6
  wires:
  Pitch2_rad/1 -> Mux2/2
  Translational Dynamics/1(E_xdot_B_E_B) -> Translational Kinematics/4(Computed V_B_E_B), V_B_E_B/1  "V_B_E_B | Velocity of Body w.r.t ECEF measured in Body"
  wBodyRates_PQR/1 -> Translational Dynamics/2(wBodyRates_PQR), Rotational Kinematics_Euler/1(wVectorBodyRates_PQR)
  Roll2_rad/1 -> Mux2/1
  Yaw2_rad/1 -> Mux2/3
  E_xdot_B_E_B_xComp/1 -> Vector Concatenate/1
  E_xdot_B_E_B_yComp/1 -> Vector Concatenate/2
  E_xdot_B_E_B_zComp/1 -> Vector Concatenate/3
  Aero Forces/1 -> Translational Dynamics/3(Aero Forces)
  Mux2/1 -> Translational Kinematics/1(Custom Attitude w.r.t ECEF)  "User Defined Attitude w.r.t ECEF"
  Rotational Kinematics_Euler/1(Theta Vector_rad) -> Translational Kinematics/2(Computed Attitude w.r.t ECEF)  "Computed Attitude w.r.t ECEF"
  Vector Concatenate/1 -> Translational Kinematics/3(Custom Body Lin Vel w.r.t ECEF)  "Custom Body Lin Vel w.r.t. ECEF"
  Translational Kinematics/1(Altitude_m) -> Altitude_m/1  "Altitude"
  Translational Kinematics/2(E_x_B_E_E) -> E_x_B_E_E/1  "Position of Body w.r.t ECEF Measured in ECEF"
  Translational Kinematics/3(C_B_N) -> Translational Dynamics/1(C_B_N), Transpose/1, C_B_N/1  "DCM from NED to Body"
  LAX Initial Pos/1 -> Translational Kinematics/5(LAX Initial Pos)
  Matrix Multiply/1 -> c_EB/1
  Transpose/1 -> Matrix Multiply/2  "C_N_B"
  Translational Kinematics/4(OutC_E_N) -> Matrix Multiply/1  "C_E_N"
  Translational Kinematics/5(position in LAX NED1) -> Position in LAX NED/1

== system ame532Project1_Gimbal_Tracking_R2022aVersion_JeosUpdates/JeoIMUmodel/Old Version/Aero Forces and Moments ==
  V_B_E_B : Inport
  C_B_N : Inport  Port=2
  F&M Horiz Stab Surface (S2) : Subsystem
  F&M Horiz Stab Surface (S3) : Subsystem
  F&M Right Wing and Servo Surface (S4) : Subsystem
  F&M Right Wing and Servo Surface (S5) : Subsystem
  Matrix Multiply : Product  Multiplication=Matrix(*)
  Sum : Sum  Inputs=|+-
  Sum1 : Sum  Inputs=|++++
  Sum2 : Sum  Inputs=|++++
  Velocity of Air Mass w.r.t. NED as measured in NED : Concatenate  NumInputs=3
  Wind in Down Direction : Constant  Value=0
  Wind in East Direction : Constant  Value=0
  Wind in North Direction : Constant  Value=20
  Mext_B : Outport
  Fext_B : Outport  Port=2
  wires:
  V_B_E_B/1 -> F&M Right Wing and Servo Surface (S5)/1(v_B_E_B), F&M Right Wing and Servo Surface (S4)/1(v_B_E_B), F&M Horiz Stab Surface (S2)/1(v_B_E_B), F&M Horiz Stab Surface (S3)/1(v_B_E_B), Sum/1
  Velocity of Air Mass w.r.t. NED as measured in NED/1 -> Matrix Multiply/2  "V_A_N_N"
  Wind in North Direction/1 -> Velocity of Air Mass w.r.t. NED as measured in NED/1
  Wind in East Direction/1 -> Velocity of Air Mass w.r.t. NED as measured in NED/2
  Wind in Down Direction/1 -> Velocity of Air Mass w.r.t. NED as measured in NED/3
  Sum/1 -> F&M Horiz Stab Surface (S2)/2(V_B_A_B (Relative AIr Speed)), F&M Horiz Stab Surface (S3)/2(V_B_A_B (Relative AIr Speed)), F&M Right Wing and Servo Surface (S5)/2(V_B_A_B (Relative AIr Speed)), F&M Right Wing and Servo Surface (S4)/2(V_B_A_B (Relative AIr Speed))  "V_B_A_B (Relative AIr Speed)"
  F&M Horiz Stab Surface (S2)/2(LiftAndDragForceS2_B) -> Sum1/1
  F&M Horiz Stab Surface (S3)/2(LiftAndDragForceS3_B) -> Sum1/2
  F&M Right Wing and Servo Surface (S4)/2(LiftAndDragForceS4_B) -> Sum1/3
  F&M Right Wing and Servo Surface (S5)/2(LiftAndDragForceS5_B) -> Sum1/4
  Sum1/1 -> Fext_B/1
  F&M Horiz Stab Surface (S2)/1(momS2_B) -> Sum2/1
  F&M Horiz Stab Surface (S3)/1(momS3_B) -> Sum2/2
  F&M Right Wing and Servo Surface (S4)/1(momS4_B) -> Sum2/3
  F&M Right Wing and Servo Surface (S5)/1(momS5_B) -> Sum2/4
  Sum2/1 -> Mext_B/1
  C_B_N/1 -> Matrix Multiply/1
  Matrix Multiply/1 -> Sum/2  "V_A_N_B"

== system ame532Project1_Gimbal_Tracking_R2022aVersion_JeosUpdates/JeoIMUmodel/Old Version/Rotational Dynamics ==
  wVector Body Rates_PQR : Inport
  Aero Moment : Inport  Port=2
  Invert 3x3 Matrix : aerolibutil/Invert  3x3 Matrix
  Jmat : sharedutil/Create 3x3 Matrix  aMode=aMode
  Jxx : Constant  Value=Jxx
  Jxy : Constant  Value=Jxy
  Jxz : Constant  Value=Jxz
  Jyx : Constant  Value=Jyx
  Jyy : Constant  Value=Jyy
  Jyz : Constant  Value=Jyz
  Jzx : Constant  Value=Jzx
  Jzy : Constant  Value=Jzy
  Jzz : Constant  Value=Jzz
  Manual Switch : ManualSwitch
  Manual Switch1 : ManualSwitch  CurrentSetting=0
  Matrix Multiply2 : Product  Multiplication=Matrix(*)
  Pitch Body Moment : Constant  Value=MM
  Roll Body Moment : Constant  Value=LL
  Sum : Sum  Inputs=|+-
  Using Cross Product Matrix : Subsystem
  Using Cross Product Operator Only : Subsystem
  Vector Concatenate : Concatenate  NumInputs=3
  Yaw Body Moment : Constant  Value=NN
  wdotVector Body Rates_PQR : Outport
  wires:
  wVector Body Rates_PQR/1 -> Using Cross Product Operator Only/1(wPQR), Using Cross Product Matrix/1(wPQR)
  Jmat/1 -> Using Cross Product Matrix/2(J Matrix), Using Cross Product Operator Only/2(J Matrix), Invert 3x3 Matrix/1
  Using Cross Product Matrix/1(OmegaJw) -> Manual Switch1/1  "OmegaJw [3x1]"
  Sum/1 -> Matrix Multiply2/2
  Matrix Multiply2/1 -> wdotVector Body Rates_PQR/1
  Jxx/1 -> Jmat/1
  Jxy/1 -> Jmat/2
  Jxz/1 -> Jmat/3
  Jyx/1 -> Jmat/4
  Jyy/1 -> Jmat/5
  Jyz/1 -> Jmat/6
  Jzx/1 -> Jmat/7
  Jzy/1 -> Jmat/8
  Jzz/1 -> Jmat/9
  Invert 3x3 Matrix/1 -> Matrix Multiply2/1  "Jinv"
  Roll Body Moment/1 -> Vector Concatenate/1
  Pitch Body Moment/1 -> Vector Concatenate/2
  Yaw Body Moment/1 -> Vector Concatenate/3
  Vector Concatenate/1 -> Manual Switch/2  "Mext_B"
  Aero Moment/1 -> Manual Switch/1
  Manual Switch/1 -> Sum/1
  Manual Switch1/1 -> Sum/2
  Using Cross Product Operator Only/1(OmegaJw) -> Manual Switch1/2

== system ame532Project1_Gimbal_Tracking_R2022aVersion_JeosUpdates/JeoIMUmodel/Old Version/Rotational Kinematics_Quaternions ==
  wVectorBodyRates_PQR : Inport
  Constant : Constant  Value=0
  Gain : Gain  Gain=0.5
  Integrator : Integrator
  Mux : Mux  Inputs=3
  NormalizeQuaternion : MATLAB Function  TreatAsAtomicUnit=on
  Quaternion Multiplication : aerolibutil/Quaternion Multiplication
  Vector Concatenate : Concatenate
  quaternionMultiplication : MATLAB Function  Commented=on  TreatAsAtomicUnit=on
  quaternionToeuler : MATLAB Function  TreatAsAtomicUnit=on
  Theta Vector_deg : Outport
  wires:
  wVectorBodyRates_PQR/1 -> Gain/1
  Gain/1 -> Vector Concatenate/2
  Constant/1 -> Vector Concatenate/1
  Integrator/1 -> NormalizeQuaternion/1(qin), quaternionToeuler/1(qin)  "q_B_N"
  quaternionToeuler/3(roll_deg) -> Mux/1
  quaternionToeuler/2(pitch_deg) -> Mux/2
  quaternionToeuler/1(yaw_deg) -> Mux/3
  NormalizeQuaternion/1(qoutNorm) -> Quaternion Multiplication/1  "q_B_N"
  Mux/1 -> Theta Vector_deg/1
  Quaternion Multiplication/1 -> Integrator/1
  Vector Concatenate/1 -> Quaternion Multiplication/2

== system ame532Project1_Gimbal_Tracking_R2022aVersion_JeosUpdates/JeoIMUmodel/Old Version/Rotational Kinematics_Strapdown ==
  wVectorBodyRates_PQR : Inport
  Demux : Demux  Outputs=3
  Integrator : Integrator
  MatrixMultiply : Product  Multiplication=Matrix(*)
  Mux : Mux  Inputs=3
  Omega_B_N : MATLAB Function  TreatAsAtomicUnit=on
  dcmTOeuler : MATLAB Function  TreatAsAtomicUnit=on
  Theta Vector_deg : Outport
  wires:
  wVectorBodyRates_PQR/1 -> Demux/1
  Demux/1 -> Omega_B_N/1(P_degPs)
  Demux/2 -> Omega_B_N/2(Q_degPs)
  Demux/3 -> Omega_B_N/3(R_degPs)
  Omega_B_N/1(y) -> MatrixMultiply/1  "omega_B_N"
  MatrixMultiply/1 -> Integrator/1  "cdot_N_B"
  Integrator/1 -> MatrixMultiply/2, dcmTOeuler/1(inputDCM)  "c_N_B"
  dcmTOeuler/3(roll_deg) -> Mux/1
  dcmTOeuler/2(pitch_deg) -> Mux/2
  dcmTOeuler/1(yaw_deg) -> Mux/3
  Mux/1 -> Theta Vector_deg/1  "Theta Vector_deg"

== system ame532Project1_Gimbal_Tracking_R2022aVersion_JeosUpdates/JeoIMUmodel/Old Version/TransKin_RotKin_TansDynam ==
  wBodyRates_PQR : Inport
  Aero Forces : Inport  Port=2
  LAx Inital Pos : Inport  Port=3
  E_xdot_B_E_B_xComp : Constant  Value=150
  E_xdot_B_E_B_yComp : Constant  Value=0
  E_xdot_B_E_B_zComp : Constant  Value=0
  Matrix Multiply : Product  Multiplication=Matrix(*)
  Mux2 : Mux  Inputs=3
  Pitch2_rad : Constant  Value=0
  Roll2_rad : Constant  Value=0
  Rotational Kinematics_Euler : Subsystem
  Translational Dynamics : Subsystem
  Translational Kinematics : Subsystem
  Transpose : Math  Operator=transpose
  Vector Concatenate : Concatenate  NumInputs=3
  Yaw2_rad : Constant  Value=0
  Altitude_m : Outport
  E_x_B_E_E : Outport  Port=2
  V_B_E_B : Outport  Port=3
  C_B_N : Outport  Port=4
  c_EB : Outport  Port=5
  position in LAX NED : Outport  Port=6
  wires:
  Pitch2_rad/1 -> Mux2/2
  Translational Dynamics/1(E_xdot_B_E_B) -> Translational Kinematics/4(Computed V_B_E_B), V_B_E_B/1  "V_B_E_B | Velocity of Body w.r.t ECEF measured in Body"
  wBodyRates_PQR/1 -> Translational Dynamics/2(wBodyRates_PQR), Rotational Kinematics_Euler/1(wVectorBodyRates_PQR)
  Roll2_rad/1 -> Mux2/1
  Yaw2_rad/1 -> Mux2/3
  E_xdot_B_E_B_xComp/1 -> Vector Concatenate/1
  E_xdot_B_E_B_yComp/1 -> Vector Concatenate/2
  E_xdot_B_E_B_zComp/1 -> Vector Concatenate/3
  Aero Forces/1 -> Translational Dynamics/3(Aero Forces)
  Mux2/1 -> Translational Kinematics/1(Custom Attitude w.r.t ECEF)  "User Defined Attitude w.r.t ECEF"
  Rotational Kinematics_Euler/1(Theta Vector_rad) -> Translational Kinematics/2(Computed Attitude w.r.t ECEF)  "Computed Attitude w.r.t ECEF"
  Vector Concatenate/1 -> Translational Kinematics/3(Custom Body Lin Vel w.r.t ECEF)  "Custom Body Lin Vel w.r.t. ECEF"
  Translational Kinematics/1(Altitude_m) -> Altitude_m/1  "Altitude"
  Translational Kinematics/2(E_x_B_E_E) -> E_x_B_E_E/1  "Position of Body w.r.t ECEF Measured in ECEF"
  Translational Kinematics/3(C_B_N) -> Transpose/1, Translational Dynamics/1(C_B_N), C_B_N/1  "DCM from NED to Body"
  LAx Inital Pos/1 -> Translational Kinematics/5(LAX Inital Pos)
  Matrix Multiply/1 -> c_EB/1
  Transpose/1 -> Matrix Multiply/2  "c_N_B"
  Translational Kinematics/4(OutC_E_N) -> Matrix Multiply/1  "C_E_N"
  Translational Kinematics/5(position in LAX NED) -> position in LAX NED/1

== system ame532Project1_Gimbal_Tracking_R2022aVersion_JeosUpdates/JeoIMUmodel/New Version/Aero Forces and Moments/F&M Horiz Stab Surface (S2) ==
  v_B_E_B : Inport
  V_B_A_B (Relative AIr Speed) : Inport  Port=2
  Compute Aero Lift and Drag : MATLAB Function  TreatAsAtomicUnit=on
  Compute Aero Moment : MATLAB Function  TreatAsAtomicUnit=on
  Constant : Constant  Value=[AR_s2 i_s2 CL0_s2 CD0_s2 CDa_s2 a0_s2 e_s2 ro area_s2]
  Constant1 : Constant  Value=[CM0_s2; CMa_s2; c_s2]
  Demux : Demux  Outputs=9
  Demux1 : Demux  Outputs=3
  F&M in Body : Subsystem
  n_s2 : Constant  Value=n_s2
  momS2_B : Outport
  LiftAndDragForceS2_B : Outport  Port=2
  wires:
  Compute Aero Lift and Drag/2(liftSurf) -> F&M in Body/2(Lift)  "Lift Force w.r.t Wind"
  Compute Aero Moment/1(momSurf) -> F&M in Body/1(momSurf)  "Moment of Surface w.r.t Wind"
  Compute Aero Lift and Drag/3(dragSurf) -> F&M in Body/3(Drag)  "Drag Force w.r.t Wind"
  F&M in Body/2(LiftAndDragForceS2_B) -> LiftAndDragForceS2_B/1
  Compute Aero Lift and Drag/1(alphaLocal) -> Compute Aero Moment/2(alphaLocal)
  v_B_E_B/1 -> Compute Aero Moment/1(v_B_E_B)
  F&M in Body/1(momS2_B) -> momS2_B/1
  V_B_A_B (Relative AIr Speed)/1 -> Compute Aero Lift and Drag/1(v_B_A_B), F&M in Body/4(v_B_A_B)
  Constant/1 -> Demux/1
  Demux/1 -> Compute Aero Lift and Drag/2(AR_s2)  "AR_s2"
  Demux/2 -> Compute Aero Lift and Drag/3(i_s2)  "i_s2"
  Demux/3 -> Compute Aero Lift and Drag/5(CL0_s2)  "CL0_s2"
  Demux/4 -> Compute Aero Lift and Drag/6(CD0_s2)  "CD0_s2"
  Demux/5 -> Compute Aero Lift and Drag/7(CDa_s2)  "CDa_s2"
  Demux/6 -> Compute Aero Lift and Drag/8(a0_s2)  "a0_s2"
  Demux/7 -> Compute Aero Lift and Drag/9(e_s2)  "e_s2"
  Demux/8 -> Compute Aero Moment/5(ro), Compute Aero Lift and Drag/10(ro)  "ro"
  Demux/9 -> Compute Aero Moment/6(area_s2), Compute Aero Lift and Drag/11(area_s2)  "area_s2"
  Constant1/1 -> Demux1/1
  Demux1/1 -> Compute Aero Moment/3(CM0_s2)  "CMo_s2"
  Demux1/2 -> Compute Aero Moment/4(CMa_s2)  "CMa_s2"
  Demux1/3 -> Compute Aero Moment/7(c_s2)  "c_s2"
  n_s2/1 -> F&M in Body/5(n_s2), Compute Aero Lift and Drag/4(n_s2)
